simulink model "work3"  (R2020b)
settings: Solver=VariableStepAuto  StartTime=0.0  StopTime=10.0  RelTol=1e-3
model workspace (MAT data in the model file):
  k = 1
settings Model: Creator=99003178  LastModifiedBy=99003178

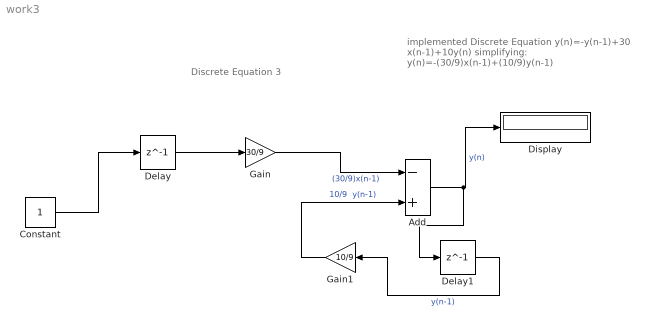
== system work3 ==
  note: Discrete Equation 3
  note: implemented Discrete Equation
      | y(n)=-y(n-1)+30 x(n-1)+10y(n)
      | simplifying:
      | y(n)=-(30/9)x(n-1)+(10/9)y(n-1)
  Add : Sum  Inputs=-+
  Constant : Constant
  Delay : Delay  DelayLength=1
  Delay1 : Delay  DelayLength=1
  Display : Display
  Gain : Gain  Gain=30/9
  Gain1 : Gain  Gain=10/9
  wires:
  Delay/1 -> Gain/1
  Gain/1 -> Add/1  "(30/9)x(n-1)"
  Add/1 -> Delay1/1, Display/1  "y(n)"
  Gain1/1 -> Add/2  "10/9  y(n-1)"
  Constant/1 -> Delay/1
  Delay1/1 -> Gain1/1  "y(n-1)"
